simulink model "FIR_fda_block"  (R2015b)
settings: Solver=FixedStepDiscrete  SolverMode=SingleTasking  StartTime=0.0  StopTime=10000/1e6  RelTol=1e-3
libraries: simulink x1
settings Model: Creator=at-mt  LastModifiedBy=amatsumo
settings DataIOCC: SaveFormat=Array  SignalLoggingSaveFormat=ModelDataLogs  SaveOutput=off  SignalLogging=off  SaveTime=off
settings OptimizationCC: BlockReduction=off  ConditionallyExecuteInputs=off  DefaultParameterBehavior=Inlined  ExpressionDepthLimit=2147483647
settings DebuggingCC: AlgebraicLoopMsg=error  UnderspecifiedInitializationDetection=Classic  MergeDetectMultiDrivingBlocksExec=none  SolverPrmCheckMsg=warning  InheritedTsInSrcMsg=none  SingleTaskRateTransMsg=error  FcnCallInpInsideContextMsg=UseLocalSettings  StateNameClashWarn=warning
settings HardwareCC: ProdBitPerPointer=32  ProdLargestAtomicFloat=None  ProdIntDivRoundTo=Undefined  ProdEndianess=Unspecified  ProdWordSize=32  ProdHWDeviceType=ASIC/FPGA->ASIC/FPGA  ProdEqTarget=off
settings GRTTargetCC: GeneratePreprocessorConditionals=Disable all  CombineOutputUpdateFcns=off  GRTInterface=on
settings ConfigComp: CovModelRefEnable=Off  CovSFcnEnable=off

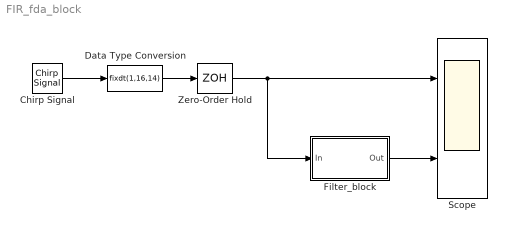
== system FIR_fda_block ==
  Chirp Signal : simulink/Sources/Chirp Signal  f1=10e3  T=10000/1e6  f2=500e3
  Data Type Conversion : DataTypeConversion  OutDataTypeStr=fixdt(1,16,14)  RndMeth=Nearest
  Filter_block : Subsystem  Tag=BlockMethodSubSystem
  Scope : Scope  NumInputPorts=2
  Zero-Order Hold : ZeroOrderHold  SampleTime=1/1e6
  wires:
  Filter_block/1(Out) -> Scope/2
  Zero-Order Hold/1 -> Filter_block/1(In), Scope/1
  Chirp Signal/1 -> Data Type Conversion/1
  Data Type Conversion/1 -> Zero-Order Hold/1

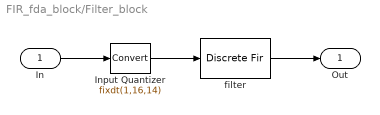
== system FIR_fda_block/Filter_block ==
  In : Inport
  Input Quantizer : DataTypeConversion  OutDataTypeStr=fixdt(1,16,14)  RndMeth=Round  SaturateOnIntegerOverflow=on
  filter : DiscreteFir  Coefficients=[-0.0015246255854119901 -0.0056040694699944459 -0.0058450039381682788 -6.2680724829390806e-05 0.0059777568571996731 0.0024746345997378864 -0.0067957421209925116 -0.0064654391449295058 0.0062328738643254028 0.011598387637803855 -0.0031016131441193155 -0.01699091246940064 -0.003469463473475945 0.021317820921314172 0.014205217299065596 -0.022739848971926518 -0.029832087938286563 0.018638954412635484 0.052011508906959603 -0.0039935685035125054 -0.087482017884039157 -0.039025075223248162 0.18476516322082137 0.40580167040079751 0.40580167040079751 0.18476516322082137 -0.039025075223248162 -0.087482017884039157 -0.0039935685035125054 0.052011508906959603 0.018638954412635484 -0.029832087938286563 -0.022739848971926518 0.014205217299065596 0.021317820921314172 -0.003469463473475945 -0.01699091246940064 -0.0031016131441193155 0.011598387637803855 0.0062328738643254028 -0.0064654391449295058 -0.0067957421209925116 0.0024746345997378864 0.0059777568571996731 -6.2680724829390806e-05 -0.0058450039381682788 -0.0056040694699944459 -0.0015246255854119901]  InputProcessing=Columns as channels (frame based)  CoefDataTypeStr=fixdt(true,16,16)  ProductDataTypeStr=fixdt(true,31,31)  AccumDataTypeStr=fixdt(true,33,31)  StateDataTypeStr=fixdt(true,33,31)  OutDataTypeStr=fixdt(true,16,14)
  Out : Outport
  wires:
  In/1 -> Input Quantizer/1
  Input Quantizer/1 -> filter/1
  filter/1 -> Out/1
